simulink model "BCI"  (Simulink 8.2)
settings: Solver=FixedStepDiscrete  StartTime=0.0  StopTime=inf  FixedStep=1/256  RelTol=1e-3
undefined symbols (not defined in the file): currentCFG_Rev_5_Experimental_Beta_Model_17_03_15_UB, UB
libraries: gRTanalyze x6, Tools x1, gUSBamplib x1
settings Model: Creator=1107941j  LastModifiedBy=abdullahg
settings DebuggingCC: MultiTaskDSMMsg=warning  MultiTaskCondExecSysMsg=none  FcnCallInpInsideContextMsg=EnableAllAsWarning
settings RTWCC: IncludeERTFirstTime=on
settings GRTTargetCC: CodeReplacementLibrary=None  CombineOutputUpdateFcns=on  CPPClassGenCompliant=on  GRTInterface=off

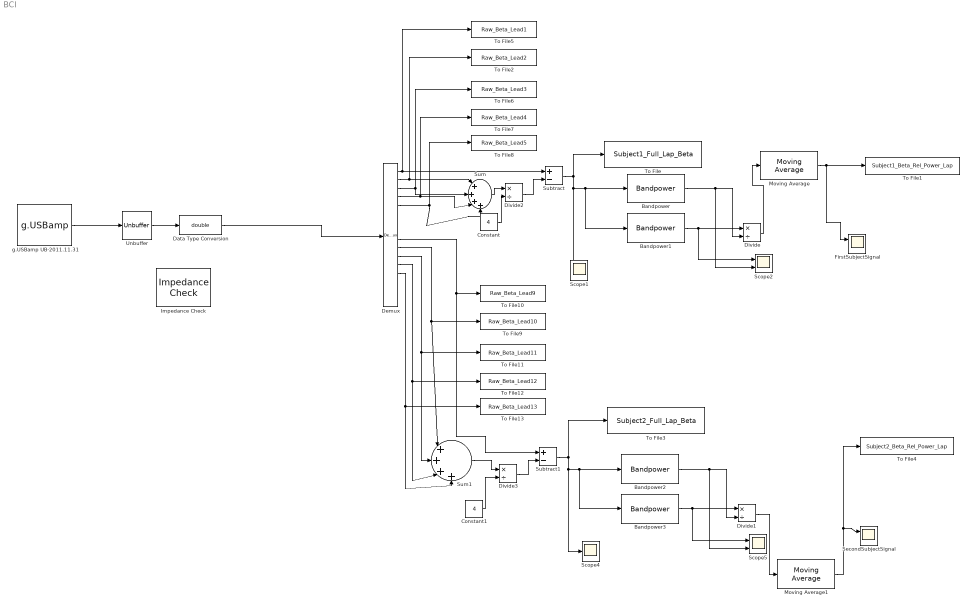
== system BCI ==
  Bandpower : gRTanalyze/Bandpower  Order=5  LowerFreq=12  UpperFreq=30  WindowLength=128
  Bandpower1 : gRTanalyze/Bandpower  Order=5  LowerFreq=5  UpperFreq=30  WindowLength=128
  Bandpower2 : gRTanalyze/Bandpower  Order=5  LowerFreq=12  UpperFreq=30  WindowLength=128
  Bandpower3 : gRTanalyze/Bandpower  Order=5  LowerFreq=5  UpperFreq=30  WindowLength=128
  Constant : Constant  Value=4
  Constant1 : Constant  Value=4
  Data Type Conversion : DataTypeConversion  OutDataTypeStr=double
  Demux : Demux  Outputs=16
  Divide{,1..3} (4 alike) : Product  Inputs=*/
  FirstSubjectSignal : Scope  NumInputPorts=2
      settings: YMin=1.5~-1  YMax=2.55~1
  Impedance Check : Tools/Impedance Check  SystemSampleTime=-1
  Moving Average : gRTanalyze/Moving Average  windowSize=256
  Moving Average1 : gRTanalyze/Moving Average  windowSize=256
  Scope1 : Scope
      settings: TimeRange=10  YMin=-60  YMax=70
  Scope2 : Scope  NumInputPorts=2
      settings: YMin=2.77556e-17~0  YMax=0.7~4.25  SaveName=ScopeData2
  Scope4 : Scope
      settings: TimeRange=10  YMin=-60  YMax=70  SaveName=ScopeData4
  Scope5 : Scope  NumInputPorts=2
      settings: YMin=2.77556e-17~0  YMax=0.7~4.25  SaveName=ScopeData5
  SecondSubjectSignal : Scope  NumInputPorts=2
      settings: YMin=1.25~-1  YMax=4.25~1  SaveName=ScopeData3
  Subtract : Sum  Inputs=+-
  Subtract1 : Sum  Inputs=+-
  Sum : Sum  Inputs=|++++
  Sum1 : Sum  Inputs=|++++
  To File : ToFile  Filename=Subject1_Full_Lap_Beta  MatrixName=Subject1_Full_Lap_Beta
  To File1 : ToFile  Filename=Subject1_Beta_Rel_Power_Lap  MatrixName=Subject1_Beta_Rel_Power_Lap
  To File10 : ToFile  Filename=Raw_Beta_Lead9  MatrixName=Raw_Beta_Lead9
  To File11 : ToFile  Filename=Raw_Beta_Lead11  MatrixName=Raw_Beta_Lead11
  To File12 : ToFile  Filename=Raw_Beta_Lead12  MatrixName=Raw_Beta_Lead12
  To File13 : ToFile  Filename=Raw_Beta_Lead13  MatrixName=Raw_Beta_Lead13
  To File2 : ToFile  Filename=Raw_Beta_Lead2  MatrixName=Raw_Beta_Lead2
  To File3 : ToFile  Filename=Subject2_Full_Lap_Beta  MatrixName=Subject2_Full_Lap_Beta
  To File4 : ToFile  Filename=Subject2_Beta_Rel_Power_Lap  MatrixName=Subject2_Beta_Rel_Power_Lap
  To File5 : ToFile  Filename=Raw_Beta_Lead1  MatrixName=Raw_Beta_Lead1
  To File6 : ToFile  Filename=Raw_Beta_Lead3  MatrixName=Raw_Beta_Lead3
  To File7 : ToFile  Filename=Raw_Beta_Lead4  MatrixName=Raw_Beta_Lead4
  To File8 : ToFile  Filename=Raw_Beta_Lead5  MatrixName=Raw_Beta_Lead5
  To File9 : ToFile  Filename=Raw_Beta_Lead10  MatrixName=Raw_Beta_Lead10
  Unbuffer : Unbuffer  SampleBasedProcessing=Same as frame based
  g.USBamp UB-2011.11.31 : gUSBamplib/g.USBamp  Priority=1  cfg=currentCFG_Rev_5_Experimental_Beta_Model_17_03_15_UB-2011.11.31.cfg  snr=UB-2011.11.31
  wires:
  g.USBamp UB-2011.11.31/1 -> Unbuffer/1
  Unbuffer/1 -> Data Type Conversion/1
  Data Type Conversion/1 -> Demux/1
  Bandpower1/1 -> Divide/1, Scope2/1
  Bandpower/1 -> Divide/2, Scope2/2
  Demux/5 -> Sum/4, To File8/1
  Demux/4 -> Sum/3, To File7/1
  Demux/3 -> To File6/1, Sum/2
  Demux/2 -> To File2/1, Sum/1
  Sum/1 -> Divide2/1
  Constant/1 -> Divide2/2
  Divide2/1 -> Subtract/2
  Demux/1 -> To File5/1, Subtract/1
  Subtract/1 -> Bandpower/1, Bandpower1/1, Scope1/1, To File/1
  Bandpower3/1 -> Divide1/1, Scope5/1
  Bandpower2/1 -> Divide1/2, Scope5/2
  Sum1/1 -> Divide3/1
  Constant1/1 -> Divide3/2
  Divide3/1 -> Subtract1/2
  Subtract1/1 -> Bandpower2/1, Bandpower3/1, Scope4/1, To File3/1
  Demux/11 -> To File11/1, Sum1/2
  Demux/9 -> To File10/1, Subtract1/1
  Demux/10 -> To File9/1, Sum1/1
  Demux/12 -> To File12/1, Sum1/3
  Demux/13 -> To File13/1, Sum1/4
  Divide/1 -> Moving Average/1
  Moving Average/1 -> FirstSubjectSignal/1, To File1/1
  Moving Average1/1 -> To File4/1, SecondSubjectSignal/1
  Divide1/1 -> Moving Average1/1
